simulink model "op_amp"  (Simulink 7.4)
settings: Solver=ode45  StartTime=0.0  StopTime=1e-5  MaxStep=1e-8  RelTol=1e-3
libraries: powerlib x7, simulink x1, simpower_extensions_1 x1
settings Model: Creator=dbenson  LastModifiedBy=Dick
settings DataIOCC: SignalLoggingName=sigsOut
settings OptimizationCC: InlineInvariantSignals=on  InitFltsAndDblsToZero=on
settings DebuggingCC: SaveWithParameterizedLinksMsg=none  SignalResolutionControl=TryResolveAllWithWarning  SolverPrmCheckMsg=none  MultiTaskDSMMsg=warning  MultiTaskCondExecSysMsg=none  StrictBusMsg=None
settings HardwareCC: TargetUnknown=on
settings RTWCC: IncludeERTFirstTime=on
settings GRTTargetCC: TargetFcnLib=ansi_tfl_tmw.mat

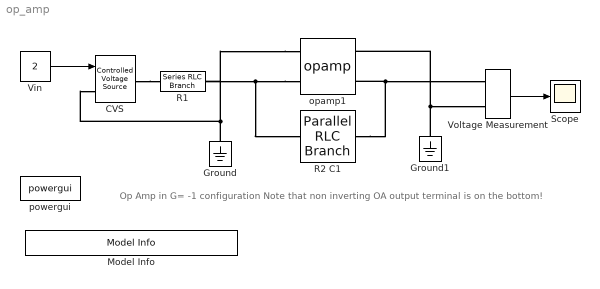
== system op_amp ==
  note: Op Amp in G= -1 configuration
      | Note that non inverting OA output terminal is on the bottom!
  CVS : powerlib/Electrical Sources/Controlled Voltage Source  Description=source block  DialogController=POWERSYS.PowerSysDialog  SystemSampleTime=-1  Initialize=off  Source_Type=AC  Amplitude=0  Phase=0  Frequency=0  Measurements=None
      settings: AttributesFormatString=\n
  Ground : powerlib/Elements/Ground  DialogController=POWERSYS.PowerSysDialog  PhysicalDomain=powersysdomain  SubClassName=unknown  LeftPortType=p1  RightPortType=p1  LConnTagsString=a
  Ground1 : powerlib/Elements/Ground  DialogController=POWERSYS.PowerSysDialog  PhysicalDomain=powersysdomain  SubClassName=unknown  LeftPortType=p1  RightPortType=p1  LConnTagsString=a
  Model Info : simulink/Model-Wide Utilities/Model Info  SystemSampleTime=-1  InitialBlockCM=None  BlockCM=None  Frame=on  DisplayStringWithTags=Copywrite 2005-2010 The MathWorks, Inc.  HorizontalTextAlignment=Center  LeftAlignmentValue=0.5  SourceBlockDiagram=op_amp  TagMaxNumber=20
  R1 : powerlib/Elements/Series RLC Branch  DialogController=POWERSYS.PowerSysDialog  PhysicalDomain=powersysdomain  SubClassName=unknown  LeftPortType=p1  RightPortType=p1  LConnTagsString=__new0  RConnTagsString=__new0  BranchType=R  Resistance=1000  Inductance=1.0  SetiL0=off  InitialCurrent=0  Capacitance=1.0  Setx0=off  InitialVoltage=0  Measurements=None
  R2 C1 : powerlib/Elements/Parallel RLC Branch  DialogController=POWERSYS.PowerSysDialog  PhysicalDomain=powersysdomain  SubClassName=unknown  LeftPortType=p1  RightPortType=p1  LConnTagsString=a  RConnTagsString=__new0  BranchType=RC  Resistance=1000  Inductance=1.0  SetiL0=off  InitialCurrent=0  Capacitance=200e-12  Setx0=off  InitialVoltage=0  Measurements=None
  Scope : Scope
      settings: TimeRange=1.2e-005  YMin=-3  YMax=0
  Vin : Constant  Value=2  OutDataType=sfix(16)  OutScaling=2^0
  Voltage Measurement : powerlib/Measurements/Voltage Measurement  Tag=PoWeRsYsTeMmEaSuReMeNt  DialogController=POWERSYS.PowerSysDialog  SystemSampleTime=-1  PhasorSimulation=off  OutputType=Magnitude  PSBequivalent=0
  opamp1 : simpower_extensions_1/opamp  SystemSampleTime=-1  f2=1e5  f1=1e4  Av=1000  v_min=-3  v_max=3  slew_rate=2e9
  powergui : powerlib/powergui  SystemSampleTime=-1  SimulationMode=Continuous  SampleTime=0  frequency=60  SPID=off  DisableSnubberDevices=off  DisableRonSwitches=off  DisableVfSwitches=off  SwTol=0  Interpol=off  frequencyindice=0  echomessages=off  HookPort=off  DisplayEquations=off  FunctionMessages=off  EnableUseOfTLC=off  x0status=blocks  RestoreLinks=warning  Frange=[0:2:500]  Ylog=off  Xlog=on  ShowGrid=off  save=off  variable=ZData  ZoomFFT=on  StartTime=0.0  cycles=1  DisplayStyle=1  fundamental=60  FreqAxis=off  MaxFrequency=1000  frequencyindicesteady=1  RmsSteady=1  display=off  Ts=0  methode=off
  wires:
  Vin/1 -> CVS/1
  Voltage Measurement/1 -> Scope/1
  connections:
  opamp1/LConn2 -- R1/RConn1 -- R2 C1/LConn1
  opamp1/LConn1 -- Ground/LConn1 -- CVS/LConn1
  opamp1/RConn2 -- R2 C1/RConn1 -- Voltage Measurement/LConn1
  opamp1/RConn1 -- Ground1/LConn1 -- Voltage Measurement/LConn2
  CVS/RConn1 -- R1/LConn1
